simulink model "old_quadSimulinkRetroComp17"  (R2017a)
settings: Solver=FixedStepAuto  StartTime=0.0  StopTime=3  FixedStep=0.005
values from neighbouring files (symbols this model uses):
  d = 2.4*10^-3    (= 0.0024)    [ScrValBackup.m]    (also in corke_plot.m = quad.d)
  dx0 = 0    [ScrValBackup.m]
  dy0 = 0    [ScrValBackup.m]
  dz0 = 0    [ScrValBackup.m]
  g = 9.81    [ScrValBackup.m]
  kr = 0.1    [ScrValBackup.m]
  l = 0.255    [ScrValBackup.m]
  m = 0.5    [ScrValBackup.m]
  p0 = 0    [ScrValBackup.m]
  phi0 = 0    [ScrValBackup.m]
  psi0 = 0.1    [ScrValBackup.m]
  q0 = 0    [ScrValBackup.m]
  r0 = 0.1177    [ScrValBackup.m]
  theta0 = 0    [ScrValBackup.m]
  x0 = 1    [ScrValBackup.m]    (also in corke_dynamics.m = init; corke_plot.m = [])
  x_coeff = A^-1*x_constr    [ScrValBackup.m]
  y0 = 1    [ScrValBackup.m]
  y_coeff = A^-1*y_constr    [ScrValBackup.m]
  z0 = 1    [ScrValBackup.m]
  z_coeff = A^-1*z_constr    [ScrValBackup.m]
undefined symbols (not defined in the file or in its folder): clientID
libraries: aerolibutil x1
settings Model: Creator=gianl  LastModifiedBy=dinies33
settings SolverCC: ZeroCrossAlgorithm=Adaptive  AlgebraicLoopSolver=LineSearch
settings DataIOCC: ReturnWorkspaceOutputs=on
settings OptimizationCC: EfficientMapNaN2IntZero=off
settings DebuggingCC: ReadBeforeWriteMsg=DisableAll  WriteAfterWriteMsg=DisableAll  WriteAfterReadMsg=DisableAll  AlgebraicLoopMsg=error  MaxConsecutiveZCsMsg=none  MaskedZcDiagnostic=none  MultiTaskDSMMsg=none
settings HardwareCC: TargetBitPerLong=64  TargetBitPerPointer=64  TargetBitPerSizeT=64  TargetBitPerPtrDiffT=64  TargetLongLongMode=on  TargetIntDivRoundTo=Zero  TargetEndianess=LittleEndian  TargetWordSize=64  TargetHWDeviceType=MATLAB Host  ProdEqTarget=off
settings ModelReferenceCC: UpdateModelReferenceTargets=IfOutOfDate
settings SFSimCC: SFSimEcho=off
settings CodeAppCC: MaxIdLength=128
settings GRTTargetCC: TargetLangStandard=C89/C90 (ANSI)  CombineOutputUpdateFcns=off  GRTInterface=on

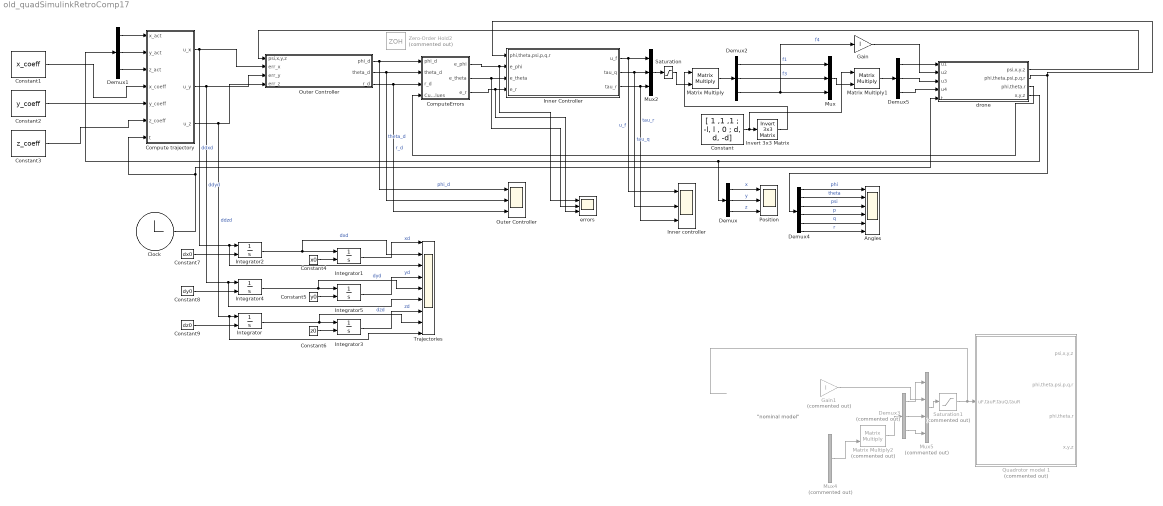
== system old_quadSimulinkRetroComp17 ==
  note: "nominal model"
  Angles : Scope  NumInputPorts=6
  Clock : Clock
  Compute trajectory : MATLAB Function  TreatAsAtomicUnit=on
  "ComputeErrors " : Subsystem
  Constant : Constant  Value=[ 1 ,1 ,1 ; -l, l , 0 ; d, d, -d]
  Constant1 : Constant  Value=x_coeff
  Constant2 : Constant  Value=y_coeff
  Constant3 : Constant  Value=z_coeff
  Constant4 : Constant  Value=x0
  Constant5 : Constant  Value=y0
  Constant6 : Constant  Value=z0
  Constant7 : Constant  Value=dx0
  Constant8 : Constant  Value=dy0
  Constant9 : Constant  Value=dz0
  Demux{,1..2,5} (4 alike) : Demux  Outputs=3
  Demux3 : Demux  Commented=on  Outputs=3
  Demux4 : Demux  Outputs=6
  Gain : Gain  Gain=l
  Gain1 : Gain  Commented=on  Gain=l
  "Inner Controller " : Subsystem
  Inner controller : Scope  NumInputPorts=3
  Integrator{,1..5} (6 alike) : Integrator  InitialConditionSource=external
  Invert 3x3 Matrix : aerolibutil/Invert  3x3 Matrix
  Matrix Multiply : Product  Multiplication=Matrix(*)
  Matrix Multiply1 : Product  Multiplication=Matrix(*)
  Matrix Multiply2 : Product  Commented=on  Multiplication=Matrix(*)
  Mux : Mux  Inputs=3
  Mux2 : Mux  Inputs=3
  Mux4 : Mux  Commented=on  Inputs=3
  Mux5 : Mux  Commented=on
  Outer Controller : Scope  NumInputPorts=3
  "Outer Controller " : Subsystem
  Position : Scope  NumInputPorts=3
  Quadrotor model 1 : Subsystem  Commented=on
  Saturation : Saturate  UpperLimit=40
  Saturation1 : Saturate  Commented=on  UpperLimit=60  LowerLimit=-60
  Trajectories : Scope  NumInputPorts=9
  Zero-Order Hold2 : ZeroOrderHold  Commented=on  SampleTime=0.1
  "drone " : Subsystem
  errors : Scope  NumInputPorts=3
  wires:
  Compute trajectory/3(u_z) -> Trajectories/9, Integrator/1, "Outer Controller "/4(err_z)  "ddzd"
  "drone "/4(x,y,z) -> Demux/1, Demux1/1
  "drone "/1("psi,x,y,z ") -> "Outer Controller "/1(psi,x,y,z)
  "drone "/2("phi,theta,psi,p,q,r ") -> "Inner Controller "/1(phi,theta,psi,p,q,r), Demux4/1
  Compute trajectory/2(u_y) -> Trajectories/6, Integrator4/1, "Outer Controller "/3(err_y)  "ddyd"
  Compute trajectory/1(u_x) -> Trajectories/3, Integrator2/1, "Outer Controller "/2(err_x)  "ddxd"
  "Inner Controller "/1(u_f) -> Inner controller/1, Mux2/1  "u_f"
  "Inner Controller "/3(tau_r) -> Inner controller/3, Mux2/3  "tau_r"
  "Inner Controller "/2(tau_q) -> Inner controller/2, Mux2/2  "tau_q"
  Constant/1 -> Matrix Multiply1/1, Invert 3x3 Matrix/1
  Invert 3x3 Matrix/1 -> Matrix Multiply/1
  Matrix Multiply/1 -> Demux2/1
  "drone "/3("phi,theta,r ") -> "ComputeErrors "/4(Curr_values)
  "ComputeErrors "/1("e_phi ") -> errors/1, "Inner Controller "/2(e_phi)
  Demux2/1 -> Mux/1  "f1"
  Demux2/2 -> Mux/2  "f3"
  Mux2/1 -> Saturation/1
  Demux1/2 -> Compute trajectory/2(y_act)
  Demux1/3 -> Compute trajectory/3(z_act)
  Constant1/1 -> Compute trajectory/4(x_coeff)
  Constant2/1 -> Compute trajectory/5(y_coeff)
  Constant3/1 -> Compute trajectory/6(z_coeff)
  Clock/1 -> "drone "/5(t), Compute trajectory/7(t)
  Demux1/1 -> Compute trajectory/1(x_act)
  "Outer Controller "/1("phi_d ") -> Outer Controller/1, "ComputeErrors "/1(phi_d)  "phi_d"
  Demux3/3 -> Mux5/4
  Mux4/1 -> Matrix Multiply2/2
  ? -> Mux4/2  "f3"
  Mux5/1 -> Saturation1/1
  Demux3/1 -> Mux5/1
  Gain1/1 -> Mux5/2
  ? -> Matrix Multiply2/1
  Saturation1/1 -> Quadrotor model 1/1(uF,tauP,tauQ,tauR)
  Matrix Multiply2/1 -> Demux3/1
  ? -> Gain1/1, Mux4/3  "f4"
  Demux3/2 -> Mux5/3
  ? -> Mux4/1  "f1"
  Integrator2/1 -> Trajectories/2, Integrator1/1  "dxd"
  Integrator1/1 -> Trajectories/1  "xd"
  Integrator/1 -> Trajectories/8, Integrator3/1  "dzd"
  Integrator4/1 -> Trajectories/5, Integrator5/1  "dyd"
  Integrator5/1 -> Trajectories/4  "yd"
  Integrator3/1 -> Trajectories/7  "zd"
  Constant7/1 -> Integrator2/2
  Constant8/1 -> Integrator4/2
  Constant9/1 -> Integrator/2
  Constant5/1 -> Integrator5/2
  Constant4/1 -> Integrator1/2
  Constant6/1 -> Integrator3/2
  "Outer Controller "/2(theta_d) -> Outer Controller/2, "ComputeErrors "/2(theta_d)  "theta_d"
  "Outer Controller "/3(r_d) -> Outer Controller/3, "ComputeErrors "/3(r_d)  "r_d"
  "ComputeErrors "/2(e_theta) -> errors/2, "Inner Controller "/3(e_theta)
  "ComputeErrors "/3(e_r) -> errors/3, "Inner Controller "/4(e_r)
  Demux/2 -> Position/2  "y"
  Demux/1 -> Position/1  "x"
  Demux/3 -> Position/3  "z"
  Demux4/1 -> Angles/1  "phi"
  Demux4/2 -> Angles/2  "theta"
  Demux4/3 -> Angles/3  "psi"
  Demux4/4 -> Angles/4  "p"
  Demux4/5 -> Angles/5  "q"
  Demux4/6 -> Angles/6  "r"
  Saturation/1 -> Matrix Multiply/2
  Demux2/3 -> Gain/1, Mux/3  "f4"
  Mux/1 -> Matrix Multiply1/2
  Demux5/1 -> "drone "/1(u1)
  Demux5/2 -> "drone "/3(u3)
  Demux5/3 -> "drone "/4(u4)
  Matrix Multiply1/1 -> Demux5/1
  Gain/1 -> "drone "/2(u2)

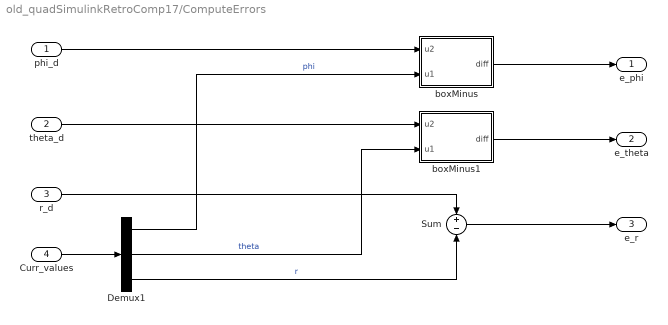
== system old_quadSimulinkRetroComp17/ComputeErrors  ==
  phi_d : Inport
  theta_d : Inport  Port=2
  r_d : Inport  Port=3
  Curr_values : Inport  Port=4
  Demux1 : Demux  Outputs=3
  Sum : Sum  Inputs=+-
  boxMinus : MATLAB Function  TreatAsAtomicUnit=on
  boxMinus1 : MATLAB Function  TreatAsAtomicUnit=on
  "e_phi " : Outport
  e_theta : Outport  Port=2
  e_r : Outport  Port=3
  wires:
  phi_d/1 -> boxMinus/1(u2)
  Demux1/1 -> boxMinus/2(u1)  "phi"
  theta_d/1 -> boxMinus1/1(u2)
  Demux1/2 -> boxMinus1/2(u1)  "theta"
  r_d/1 -> Sum/1
  Demux1/3 -> Sum/2  "r"
  Sum/1 -> e_r/1
  boxMinus1/1(diff) -> e_theta/1
  boxMinus/1(diff) -> "e_phi "/1
  Curr_values/1 -> Demux1/1

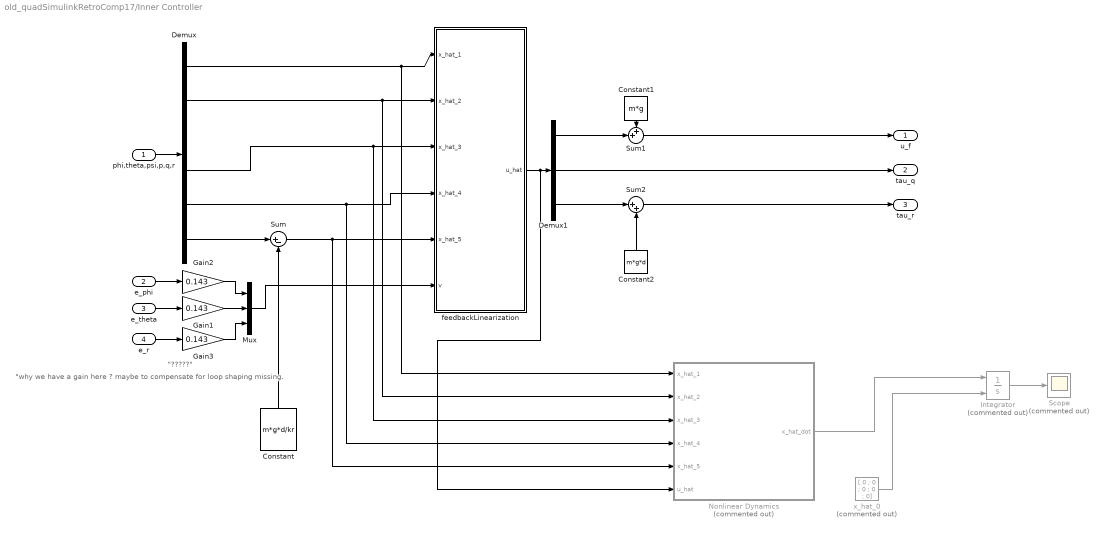
== system old_quadSimulinkRetroComp17/Inner Controller  ==
  note: "why we have a gain here ? maybe to compensate for loop shaping missing.
  note: "?????"
  phi,theta,psi,p,q,r : Inport
  e_phi : Inport  Port=2
  e_theta : Inport  Port=3
  e_r : Inport  Port=4
  Constant : Constant  Value=m*g*d/kr
  Constant1 : Constant  Value=m*g
  Constant2 : Constant  Value=m*g*d
  Demux : Demux  Outputs=6
  Demux1 : Demux  Outputs=3
  Gain1 : Gain  Gain=0.143
  Gain2 : Gain  Gain=0.143
  Gain3 : Gain  Gain=0.143
  Integrator : Integrator  Commented=on  InitialConditionSource=external
  Mux : Mux  Inputs=3
  "Nonlinear Dynamics " : MATLAB Function  Commented=on  TreatAsAtomicUnit=on
  Scope : Scope  Commented=on
  Sum : Sum  Inputs=|+-
  Sum1 : Sum  Inputs=++|
  Sum2 : Sum  Inputs=|++
  feedbackLinearization : MATLAB Function  TreatAsAtomicUnit=on
  x_hat_0 : Constant  Commented=on  Value=[ 0 ; 0 ; 0 ; 0 ; 0]
  u_f : Outport
  tau_q : Outport  Port=2
  tau_r : Outport  Port=3
  wires:
  phi,theta,psi,p,q,r/1 -> Demux/1
  Demux/1 -> feedbackLinearization/1(x_hat_1), "Nonlinear Dynamics "/1(x_hat_1)
  Demux/2 -> feedbackLinearization/2(x_hat_2), "Nonlinear Dynamics "/2(x_hat_2)
  Demux/4 -> "Nonlinear Dynamics "/3(x_hat_3), feedbackLinearization/3(x_hat_3)
  Demux/5 -> feedbackLinearization/4(x_hat_4), "Nonlinear Dynamics "/4(x_hat_4)
  e_phi/1 -> Gain2/1
  "Nonlinear Dynamics "/1(x_hat_dot) -> Integrator/1
  x_hat_0/1 -> Integrator/2
  Demux/6 -> Sum/1
  Constant/1 -> Sum/2
  Sum/1 -> "Nonlinear Dynamics "/5(x_hat_5), feedbackLinearization/5(x_hat_5)
  Demux1/3 -> Sum2/1
  Demux1/1 -> Sum1/2
  Constant1/1 -> Sum1/1
  Sum1/1 -> u_f/1
  Demux1/2 -> tau_q/1
  Constant2/1 -> Sum2/2
  Sum2/1 -> tau_r/1
  feedbackLinearization/1(u_hat) -> "Nonlinear Dynamics "/6(u_hat), Demux1/1
  Integrator/1 -> Scope/1
  e_theta/1 -> Gain1/1
  e_r/1 -> Gain3/1
  Mux/1 -> feedbackLinearization/6(v)
  Gain2/1 -> Mux/1
  Gain1/1 -> Mux/2
  Gain3/1 -> Mux/3

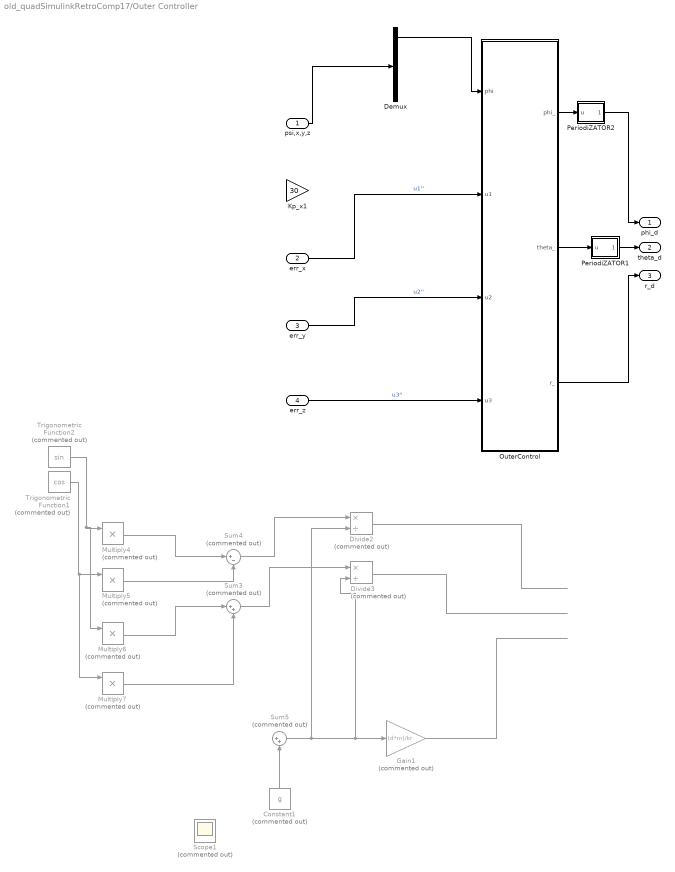
== system old_quadSimulinkRetroComp17/Outer Controller  ==
  psi,x,y,z : Inport  SampleTime=0.1
  err_x : Inport  Port=2
  err_y : Inport  Port=3
  err_z : Inport  Port=4
  Constant1 : Constant  Commented=on  Value=g
  Demux : Demux
  Divide2 : Product  Commented=on  Inputs=*/
  Divide3 : Product  Commented=on  Inputs=*/
  Gain1 : Gain  Commented=on  Gain=(d*m)/kr
  Kp_x1 : Gain  Gain=30
  Multiply{4..7} (4 alike) : Product  Commented=on
  OuterControl : MATLAB Function  TreatAsAtomicUnit=on
  PeriodiZATOR1 : MATLAB Function  TreatAsAtomicUnit=on
  PeriodiZATOR2 : MATLAB Function  TreatAsAtomicUnit=on
  Scope1 : Scope  Commented=on
  Sum3 : Sum  Commented=on  Inputs=|++
  Sum4 : Sum  Commented=on  Inputs=|+-
  Sum5 : Sum  Commented=on  Inputs=|++
  Trigonometric Function1 : Trigonometry  Commented=on  Operator=cos
  Trigonometric Function2 : Trigonometry  Commented=on
  "phi_d " : Outport
  theta_d : Outport  Port=2
  r_d : Outport  Port=3
  wires:
  psi,x,y,z/1 -> Demux/1
  Demux/1 -> OuterControl/1(phi)
  Divide2/1 -> ?
  Divide3/1 -> ?
  Gain1/1 -> ?
  Sum5/1 -> Gain1/1, Divide3/2, Divide2/2
  Constant1/1 -> Sum5/2
  Multiply6/1 -> Sum3/1
  Multiply7/1 -> Sum3/2
  Multiply5/1 -> Sum4/2
  Trigonometric Function1/1 -> Multiply5/1, Multiply7/1
  Trigonometric Function2/1 -> Multiply4/1, Multiply6/1
  Multiply4/1 -> Sum4/1
  ? -> Trigonometric Function2/1
  ? -> Trigonometric Function1/1
  ? -> Scope1/1, Sum5/1  "u3''"
  Sum3/1 -> Divide3/1
  Sum4/1 -> Divide2/1
  ? -> Multiply5/2, Multiply6/2  "u2''"
  ? -> Multiply7/2  "u1''"
  ? -> Multiply4/2  "u1''"
  err_x/1 -> OuterControl/2(u1)  "u1''"
  err_y/1 -> OuterControl/3(u2)  "u2''"
  err_z/1 -> OuterControl/4(u3)  "u3''"
  OuterControl/1(phi_) -> PeriodiZATOR2/1(u)
  OuterControl/2(theta_) -> PeriodiZATOR1/1(u)
  OuterControl/3(r_) -> r_d/1
  PeriodiZATOR2/1(angle) -> "phi_d "/1
  PeriodiZATOR1/1(angle) -> theta_d/1

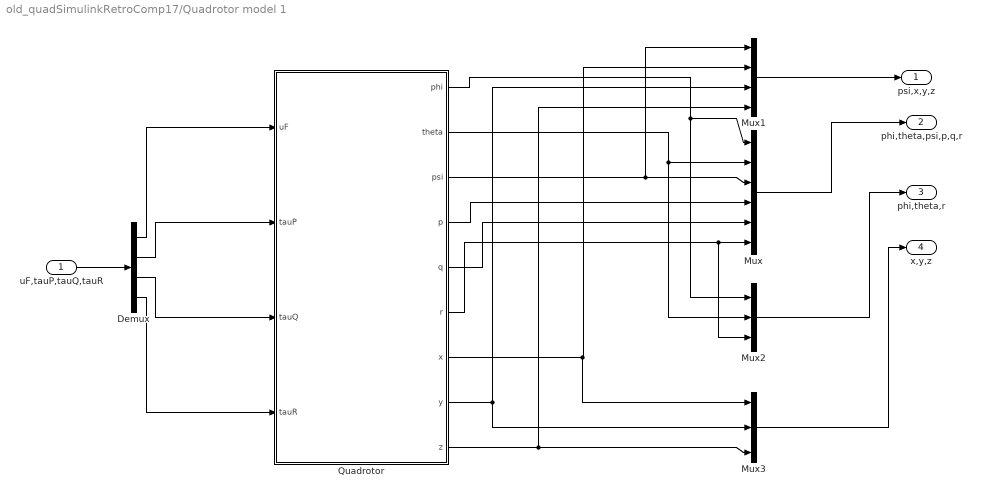
== system old_quadSimulinkRetroComp17/Quadrotor model 1 ==
  uF,tauP,tauQ,tauR : Inport
  Demux : Demux
  Mux : Mux  Inputs=6
  Mux1 : Mux
  Mux2 : Mux  Inputs=3
  Mux3 : Mux  Inputs=3
  "Quadrotor " : Subsystem
  "psi,x,y,z " : Outport
  "phi,theta,psi,p,q,r " : Outport  Port=2
  "phi,theta,r " : Outport  Port=3
  x,y,z : Outport  Port=4
  wires:
  uF,tauP,tauQ,tauR/1 -> Demux/1
  Mux1/1 -> "psi,x,y,z "/1
  Mux/1 -> "phi,theta,psi,p,q,r "/1
  Mux2/1 -> "phi,theta,r "/1
  Mux3/1 -> x,y,z/1
  "Quadrotor "/4(p) -> Mux/4
  "Quadrotor "/5(q) -> Mux/5
  "Quadrotor "/6(r) -> Mux/6, Mux2/3
  "Quadrotor "/7(x) -> Mux3/1, Mux1/2
  "Quadrotor "/8(y) -> Mux1/3, Mux3/2
  "Quadrotor "/9(z) -> Mux1/4, Mux3/3
  Demux/1 -> "Quadrotor "/1(uF)
  Demux/2 -> "Quadrotor "/2(tauP)
  Demux/3 -> "Quadrotor "/3(tauQ)
  Demux/4 -> "Quadrotor "/4(tauR)
  "Quadrotor "/1(phi) -> Mux2/1, Mux/1
  "Quadrotor "/2(theta) -> Mux2/2, Mux/2
  "Quadrotor "/3(psi) -> Mux/3, Mux1/1

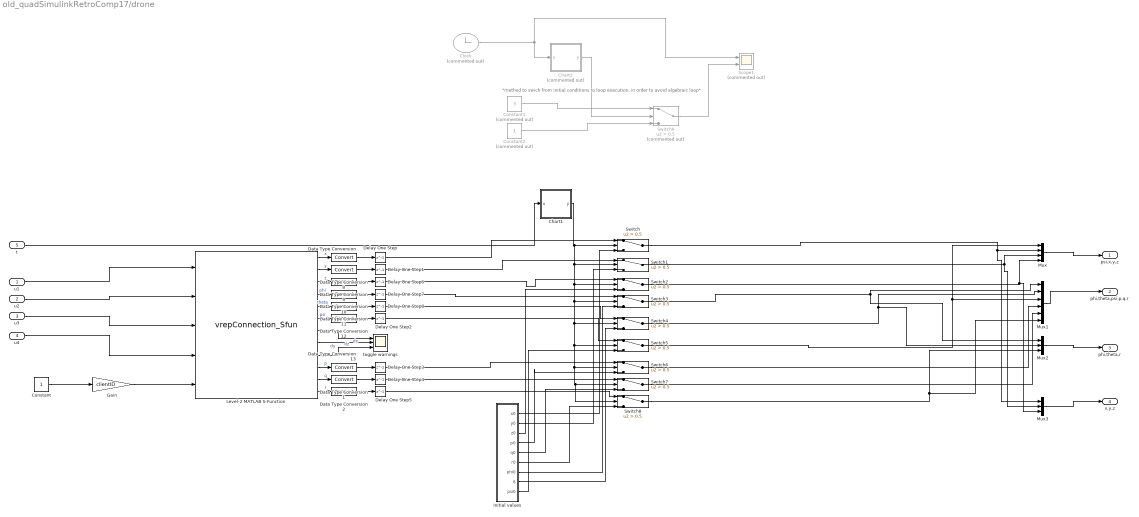
== system old_quadSimulinkRetroComp17/drone  ==
  note: "method to swich from initial conditions to loop execution, in order to avoid algebraic loop"
  u1 : Inport
  u2 : Inport  Port=2
  u3 : Inport  Port=3
  u4 : Inport  Port=4
  t : Inport  Port=5
  Chart1 : Stateflow chart  TreatAsAtomicUnit=on
  Chart2 : Stateflow chart  Commented=on  TreatAsAtomicUnit=on
  Clock : Clock  Commented=on
  Constant : Constant
  Constant1 : Constant  Commented=on  Value=3
  Constant2 : Constant  Commented=on
  Data Type Conversion{,1..2,8..13} (9 alike) : DataTypeConversion
  Delay One Step{,1..8} (9 alike) : Delay  DelayLength=1
  Gain : Gain  Gain=clientID
  "Initial values " : Subsystem
  Level-2 MATLAB S-Function : M-S-Function  FunctionName=vrepConnection_Sfun
  Mux : Mux
  Mux1 : Mux  Inputs=6
  Mux2 : Mux  Inputs=3
  Mux3 : Mux  Inputs=3
  Scope1 : Scope  Commented=on  NumInputPorts=2
  Switch{,1..8} (9 alike) : Switch  Criteria=u2 > Threshold  Threshold=0.5
  Switch9 : Switch  Commented=on  Criteria=u2 > Threshold  Threshold=0.5
  toggle warnings : Scope  NumInputPorts=3
  "psi,x,y,z " : Outport
  "phi,theta,psi,p,q,r " : Outport  Port=2
  "phi,theta,r " : Outport  Port=3
  x,y,z : Outport  Port=4
  wires:
  u1/1 -> Level-2 MATLAB S-Function/1
  u2/1 -> Level-2 MATLAB S-Function/2
  u3/1 -> Level-2 MATLAB S-Function/3
  u4/1 -> Level-2 MATLAB S-Function/4
  Constant/1 -> Gain/1
  Gain/1 -> Level-2 MATLAB S-Function/5
  Level-2 MATLAB S-Function/6 -> Data Type Conversion12/1  "psi"
  Level-2 MATLAB S-Function/5 -> Data Type Conversion11/1  "theta"
  Level-2 MATLAB S-Function/4 -> Data Type Conversion10/1  "phi"
  Level-2 MATLAB S-Function/3 -> Data Type Conversion9/1  "z"
  Level-2 MATLAB S-Function/2 -> Data Type Conversion8/1  "y"
  Level-2 MATLAB S-Function/1 -> Data Type Conversion/1  "x"
  Level-2 MATLAB S-Function/12 -> Data Type Conversion2/1  "r"
  Level-2 MATLAB S-Function/11 -> Data Type Conversion1/1  "q"
  Level-2 MATLAB S-Function/10 -> Data Type Conversion13/1  "p"
  Mux3/1 -> x,y,z/1
  Mux2/1 -> "phi,theta,r "/1
  Mux/1 -> "psi,x,y,z "/1
  Mux1/1 -> "phi,theta,psi,p,q,r "/1
  Switch/1 -> Mux3/1, Mux/2
  Switch1/1 -> Mux3/2, Mux/3
  Switch2/1 -> Mux/4, Mux3/3
  Switch3/1 -> Mux2/1, Mux1/1
  Switch4/1 -> Mux1/2, Mux2/2
  Switch5/1 -> Mux/1, Mux1/3
  Switch6/1 -> Mux1/4
  Switch7/1 -> Mux1/5
  Switch8/1 -> Mux2/3, Mux1/6
  t/1 -> Chart1/1(u)
  Data Type Conversion/1 -> Delay One Step/1
  "Initial values "/1(x0) -> Switch/3
  Data Type Conversion8/1 -> Delay One Step1/1
  "Initial values "/2(y0) -> Switch1/3
  Data Type Conversion9/1 -> Delay One Step6/1
  "Initial values "/3(z0) -> Switch2/3
  Data Type Conversion10/1 -> Delay One Step7/1
  "Initial values "/7(phi0) -> Switch3/3
  "Initial values "/8(theta0) -> Switch4/3
  Data Type Conversion11/1 -> Delay One Step8/1
  Data Type Conversion12/1 -> Delay One Step2/1
  "Initial values "/9(psi0) -> Switch5/3
  Data Type Conversion13/1 -> Delay One Step3/1
  "Initial values "/4(p0) -> Switch6/3
  Data Type Conversion1/1 -> Delay One Step4/1
  "Initial values "/5(q0) -> Switch7/3
  "Initial values "/6(r0) -> Switch8/3
  Data Type Conversion2/1 -> Delay One Step5/1
  Chart2/1(y) -> Switch9/2
  Clock/1 -> Scope1/1, Chart2/1(u)
  Constant1/1 -> Switch9/1
  Switch9/1 -> Scope1/2
  Constant2/1 -> Switch9/3
  Delay One Step5/1 -> Switch8/1
  Delay One Step4/1 -> Switch7/1
  Delay One Step3/1 -> Switch6/1
  Delay One Step2/1 -> Switch5/1
  Delay One Step1/1 -> Switch1/1
  Delay One Step/1 -> Switch/1
  Delay One Step6/1 -> Switch2/1
  Delay One Step7/1 -> Switch3/1
  Delay One Step8/1 -> Switch4/1
  Chart1/1(y) -> Switch3/2, Switch8/2, Switch7/2, Switch6/2, Switch5/2, Switch4/2, Switch2/2, Switch1/2, Switch/2
  Level-2 MATLAB S-Function/7 -> toggle warnings/1  "dx"
  Level-2 MATLAB S-Function/8 -> toggle warnings/2  "dy"
  Level-2 MATLAB S-Function/9 -> toggle warnings/3  "dz"

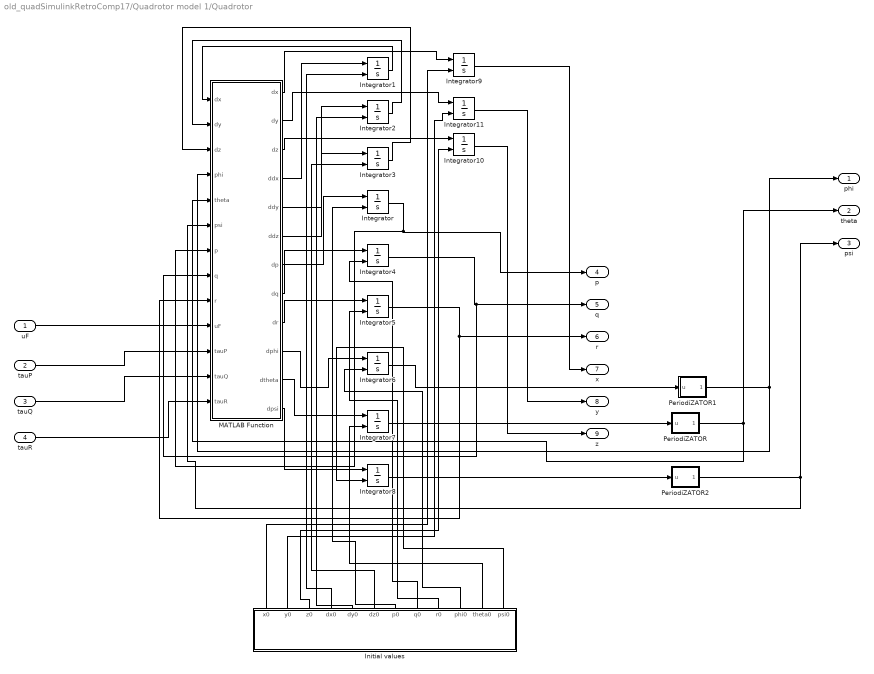
== system old_quadSimulinkRetroComp17/Quadrotor model 1/Quadrotor  ==
  uF : Inport
  tauP : Inport  Port=2
  tauQ : Inport  Port=3
  tauR : Inport  Port=4
  "Initial values " : Subsystem
  Integrator{,1..11} (12 alike) : Integrator  InitialConditionSource=external
  MATLAB Function : MATLAB Function  TreatAsAtomicUnit=on
  PeriodiZATOR : MATLAB Function  TreatAsAtomicUnit=on
  PeriodiZATOR1 : MATLAB Function  TreatAsAtomicUnit=on
  PeriodiZATOR2 : MATLAB Function  TreatAsAtomicUnit=on
  phi : Outport
  theta : Outport  Port=2
  psi : Outport  Port=3
  p : Outport  Port=4
  q : Outport  Port=5
  r : Outport  Port=6
  x : Outport  Port=7
  y : Outport  Port=8
  z : Outport  Port=9
  wires:
  uF/1 -> MATLAB Function/10(uF)
  tauP/1 -> MATLAB Function/11(tauP)
  tauQ/1 -> MATLAB Function/12(tauQ)
  tauR/1 -> MATLAB Function/13(tauR)
  MATLAB Function/12(dpsi) -> Integrator8/1
  Integrator8/1 -> PeriodiZATOR2/1(u)
  MATLAB Function/11(dtheta) -> Integrator7/1
  Integrator7/1 -> PeriodiZATOR/1(u)
  MATLAB Function/10(dphi) -> Integrator6/1
  Integrator6/1 -> PeriodiZATOR1/1(u)
  MATLAB Function/9(dr) -> Integrator5/1
  Integrator5/1 -> MATLAB Function/9(r), r/1
  MATLAB Function/8(dq) -> Integrator4/1
  Integrator4/1 -> MATLAB Function/8(q), q/1
  MATLAB Function/7(dp) -> Integrator/1
  Integrator/1 -> MATLAB Function/7(p), p/1
  MATLAB Function/6(ddz) -> Integrator3/1
  MATLAB Function/5(ddy) -> Integrator2/1
  MATLAB Function/4(ddx) -> Integrator1/1
  Integrator3/1 -> MATLAB Function/3("dz ")
  Integrator2/1 -> MATLAB Function/2("dy ")
  Integrator1/1 -> MATLAB Function/1("dx ")
  Integrator9/1 -> x/1
  Integrator11/1 -> y/1
  Integrator10/1 -> z/1
  "Initial values "/1(x0) -> Integrator9/2
  "Initial values "/2(y0) -> Integrator11/2
  "Initial values "/3(z0) -> Integrator10/2
  "Initial values "/4(dx0) -> Integrator1/2
  "Initial values "/5(dy0) -> Integrator2/2
  "Initial values "/6(dz0) -> Integrator3/2
  "Initial values "/7(p0) -> Integrator/2
  "Initial values "/8(q0) -> Integrator4/2
  "Initial values "/9(r0) -> Integrator5/2
  "Initial values "/10(phi0) -> Integrator6/2
  "Initial values "/11(theta0) -> Integrator7/2
  "Initial values "/12(psi0) -> Integrator8/2
  MATLAB Function/1(dx) -> Integrator9/1
  MATLAB Function/2(dy) -> Integrator11/1
  MATLAB Function/3(dz) -> Integrator10/1
  PeriodiZATOR/1(angle) -> theta/1, MATLAB Function/5(theta)
  PeriodiZATOR1/1(angle) -> phi/1, MATLAB Function/4(phi)
  PeriodiZATOR2/1(angle) -> psi/1, MATLAB Function/6(psi)

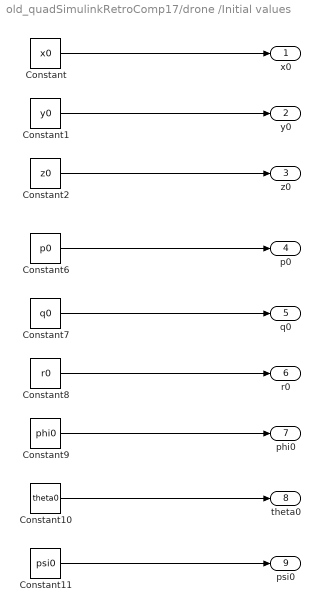
== system old_quadSimulinkRetroComp17/drone /Initial values  ==
  Constant : Constant  Value=x0
  Constant1 : Constant  Value=y0
  Constant10 : Constant  Value=theta0
  Constant11 : Constant  Value=psi0
  Constant2 : Constant  Value=z0
  Constant6 : Constant  Value=p0
  Constant7 : Constant  Value=q0
  Constant8 : Constant  Value=r0
  Constant9 : Constant  Value=phi0
  x0 : Outport
  y0 : Outport  Port=2
  z0 : Outport  Port=3
  p0 : Outport  Port=4
  q0 : Outport  Port=5
  r0 : Outport  Port=6
  phi0 : Outport  Port=7
  theta0 : Outport  Port=8
  psi0 : Outport  Port=9
  wires:
  Constant/1 -> x0/1
  Constant1/1 -> y0/1
  Constant2/1 -> z0/1
  Constant6/1 -> p0/1
  Constant7/1 -> q0/1
  Constant8/1 -> r0/1
  Constant9/1 -> phi0/1
  Constant10/1 -> theta0/1
  Constant11/1 -> psi0/1

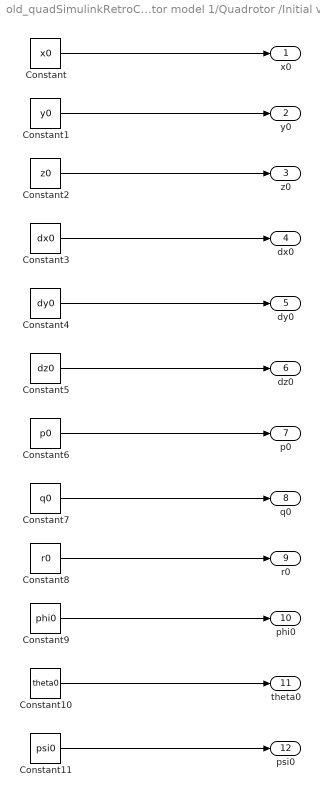
== system old_quadSimulinkRetroComp17/Quadrotor model 1/Quadrotor /Initial values  ==
  Constant : Constant  Value=x0
  Constant1 : Constant  Value=y0
  Constant10 : Constant  Value=theta0
  Constant11 : Constant  Value=psi0
  Constant2 : Constant  Value=z0
  Constant3 : Constant  Value=dx0
  Constant4 : Constant  Value=dy0
  Constant5 : Constant  Value=dz0
  Constant6 : Constant  Value=p0
  Constant7 : Constant  Value=q0
  Constant8 : Constant  Value=r0
  Constant9 : Constant  Value=phi0
  x0 : Outport
  y0 : Outport  Port=2
  z0 : Outport  Port=3
  dx0 : Outport  Port=4
  dy0 : Outport  Port=5
  dz0 : Outport  Port=6
  p0 : Outport  Port=7
  q0 : Outport  Port=8
  r0 : Outport  Port=9
  phi0 : Outport  Port=10
  theta0 : Outport  Port=11
  psi0 : Outport  Port=12
  wires:
  Constant/1 -> x0/1
  Constant1/1 -> y0/1
  Constant2/1 -> z0/1
  Constant3/1 -> dx0/1
  Constant4/1 -> dy0/1
  Constant5/1 -> dz0/1
  Constant6/1 -> p0/1
  Constant7/1 -> q0/1
  Constant8/1 -> r0/1
  Constant9/1 -> phi0/1
  Constant10/1 -> theta0/1
  Constant11/1 -> psi0/1

== matlab function old_quadSimulinkRetroComp17/Inner Controller /feedbackLinearization ==
  data: x_hat_1 input; x_hat_2 input; x_hat_3 input; x_hat_4 input; x_hat_5 input; u_hat output; v input
function u_hat= fcn(x_hat_1,x_hat_2,x_hat_3,x_hat_4,x_hat_5, v)
m= 0.5;
g= 9.81;
d= 1/2; %2.4*10^-3;
kr = 2*10^-3; %extimate for r = 6 (1 rounds /second) 
Ixx= 5.9*10-3;
Iyy= 5.9*10-3;
Izz= 1.16*10-3;
l= 0.255;

x1 = x_hat_1;
x2 = x_hat_2;
x3 = x_hat_3;
x4 = x_hat_4;
x5 = x_hat_5;

alfa = zeros(3,1);

alfa(1,1) = -2*l*Izz*kr^2*(Ixx*(-1/4*cos(x2)^-2*Izz*(2*d^2*g^2*m^2*...
    (sin(2*x1) + x1 + cos(2*x2)*(-4*sin(x1) +x1 ) -sin(2*x2)*x2*tan(x1))+...
    2*d*g*m*kr*( -3*x4 - 4*cos(2*x2)*sin(x1)*x5+ cos(x1)^-1 *(2*x4- ...
    cos(3*x1)*x4 + 2*cos(2*x1)*cos(2*x2)*x4 + sin(3*x1)*x5)+ ...
    (2*sin(2*x2)*x3+ x5)* tan(x1))+ kr^2*( -6*x4*x5 - cos(x1)^-1 *...
    (2 *sin(2*x2)*x3*x4 + 2*cos(3*x1)*x4*x5 + sin(3*x1)*(x4- x5)*(x4+x5))+...
    (x5^2 - 3*x4^2+2*cos(2*x2)*x4^2)*tan(x1))) - cos(x1)^-1*kr^3*x5*tan(x2))+...
    Izz*( kr^2*( cos(x1)^-1 *kr*x5*tan(x2) - d*g*m*( x2+ cos(x1)^-1 *(-1+...
    sin(x1)*x1)*tan(x2)))+Izz*( -kr^2 *x4*x5+d*g*m*kr*(-x4+cos(x1)*x4-...
    sin(x1)*x5+x3*tan(x1)*tan(x2)+ sin(x1)*( x5+ x4*tan(x1))*tan(x2)^2)+...
    d^2 * g^2 * m^2 * (x1- x2*tan(x1)*tan(x2)+ sin(x1)* (-1+ tan(x2)^2)))));

alfa(2,1) =  Izz*kr^2*(Ixx*(-kr^3* x5*tan(x1)+ Izz*( d^2*g^2*m^2*(cos(x1)^-1* ...
    x2 + (-2+cos(x1)) *tan(x2)) + kr^2*(x3*(2*x5+x4*tan(x1))+ cos(x1)^-1*(sin(x1)*...
    x4+ cos(x1)*x5)^2 * tan(x2)) + 2*d*g*m*kr*( x3 - cos(x1)^-1*x3+ (sin(x1)*x4- ...
    x5 +cos(x1)*x5 - x4*tan(x1))* tan(x2)))) + Izz * ( cos(x1)^-1 * kr^2*...
    (d*g*m*( sin(x1) - x1) + sin(x1)*kr*x5) + Izz *(-kr^2*x3*x5+ d^2*g^2*m^2*...
    (-cos(x1)^-1*x2 + tan(x2))+ d*g*m*kr*((-1+ cos(x1)^-1)*x3+(x5+x4*tan(x1))*...
    tan(x2)))));

alfa(3,1) = 0;

% elem 2,2 is dubious, on the paper is written as SCx1, what is S ?
beta = [
    1 , -2*(tan(x1)*tan(x2))/l , -2*(cos(x1)^-1*Ixx*tan(x2))/(l*Izz) ; 
    0 ,  sin(x1)*cos(x1) , Ixx*tan(x1)/Izz ;
    0 ,  0  ,   1;
    ];


u_hat = alfa + beta* v;

== stateflow chart old_quadSimulinkRetroComp17/drone /Chart2 ==
  state ciao
    en, du: y=0;
  state fica
    en, du: y=1;
  ciao -> fica : [u > 0]
  (default) -> ciao
  data: y output; u input

== matlab function old_quadSimulinkRetroComp17/Inner Controller /Nonlinear Dynamics  ==
  data: x_hat_1 input; x_hat_2 input; x_hat_3 input; x_hat_4 input; x_hat_5 input; x_hat_dot output; u_hat input
function x_hat_dot = fcn(x_hat_1,x_hat_2,x_hat_3,x_hat_4,x_hat_5,u_hat)

m= 0.5;
g= 9.81;
d= 2.4*10^-3;
kr = 2*10^-3; %extimate for r = 6 (1 rounds /second) 
Ixx= 5.9*10-3;
Iyy= 5.9*10-3;
Izz= 1.16*10-3;
l= 0.255;
x_hat = [x_hat_1;
        x_hat_2;
        x_hat_3;
        x_hat_4;
        x_hat_5];

f = [
    x_hat(3,1)+x_hat(4,1)*sin(x_hat(1,1))*tan(x_hat(2,1)) + ( x_hat(5,1)+ m*g*d/kr)*cos(x_hat(1,1))*tan(x_hat(2,1));
    x_hat(4,1)*cos(x_hat(1,1))- (x_hat(5,1)+ m*g*d/kr)*sin(x_hat(1,1)) ;
    1/Ixx*( -kr*x_hat(3,1)- x_hat(4,1)*(x_hat(5,1)+ m*g*d/kr)*(Izz - Ixx));
    1/Iyy*( -kr*x_hat(4,1)- x_hat(3,1)*(x_hat(5,1)+ m*g*d/kr)*(Ixx - Izz));
    1/Izz*(-kr* x_hat(5,1));    
    ];
G = [
    0 , 0 , 0;
    0,  0 , 0;
    l/(2*Ixx), 0 , -l/(2*d*Ixx)
    0,  1/Iyy  , 0 ;
    0 ,  0   ,  1/Izz;
    ];

    
x_hat_dot = f + G*u_hat;

== stateflow chart old_quadSimulinkRetroComp17/drone /Chart1 ==
  state ciao
    en, du: y=0;
  state fica
    en, du: y=1;
  ciao -> fica : [u > 0]
  (default) -> ciao
  data: y output; u input

== matlab function old_quadSimulinkRetroComp17/ComputeErrors /boxMinus ==
  data: u2 input; diff output; u1 input
function diff = fcn(u2, u1)

R2 = [cos(u2) -sin(u2);
      sin(u2) cos(u2)];

R1 = [cos(-u1) -sin(-u1);
      sin(-u1) cos(-u1)];

R = R2*R1;

diff = atan2(R(2,1), R(1,1));

== matlab function old_quadSimulinkRetroComp17/ComputeErrors /boxMinus1 ==
  data: u2 input; diff output; u1 input
function diff = fcn(u2, u1)

R2 = [cos(u2) -sin(u2);
      sin(u2) cos(u2)];

R1 = [cos(-u1) -sin(-u1);
      sin(-u1) cos(-u1)];

R = R2*R1;

diff = atan2(R(2,1), R(1,1));

== matlab function old_quadSimulinkRetroComp17/Outer Controller /PeriodiZATOR1 ==
  data: u input; angle output
function angle = fcn(u)

y = sin(u);
x = cos(u);

angle = atan2(y,x);

== matlab function old_quadSimulinkRetroComp17/Outer Controller /PeriodiZATOR2 ==
  data: u input; angle output
function angle = fcn(u)

y = sin(u);
x = cos(u);

angle = atan2(y,x);

== matlab function old_quadSimulinkRetroComp17/Compute trajectory ==
  data: x_act input; y_act input; z_act input; x_coeff input; u_x output; y_coeff input; z_coeff input; u_y output; u_z output; t input
function [u_x, u_y, u_z]  = fcn(x_act, y_act, z_act, x_coeff, y_coeff, z_coeff, t)

x_ = x_coeff(1)*t^3+x_coeff(2)*t^2+x_coeff(3)*t+x_coeff(4);
y_ = y_coeff(1)*t^3+y_coeff(2)*t^2+y_coeff(3)*t+y_coeff(4);
z_ = z_coeff(1)*t^3+z_coeff(2)*t^2+z_coeff(3)*t+z_coeff(4);

x_ddot = 6*x_coeff(1)*t+2*x_coeff(2);
y_ddot = 6*y_coeff(1)*t+2*y_coeff(2);
z_ddot = 6*z_coeff(1)*t+2*z_coeff(2);

u_x = x_ddot + 1.2*(x_ - x_act);
u_y = y_ddot + 0.9*(y_ - y_act);
u_z = z_ddot + 2.3*(z_ - z_act);

== matlab function old_quadSimulinkRetroComp17/Outer Controller /OuterControl ==
  data: phi input; phi_ output; u1 input; u2 input; u3 input; theta_ output; r_ output
function [phi_, theta_, r_] = fcn(phi, u1, u2, u3)

m= 0.5;
g= 9.81;
d= 1/2; %2.4*10^-3;
kr = 1/2; %2*10^-3; %extimate for r = 6 (1 rounds /second) 
l= 0.255;

R = [sin(phi), -cos(phi);
    cos(phi), sin(phi)];


u12 = R*[u1;u2];

u3 = u3 + g;

r_ = u3*d*m/kr;
phi_ = u12(1)/u3;
theta_ = u12(2)/u3;

== matlab function old_quadSimulinkRetroComp17/Quadrotor model 1/Quadrotor /MATLAB Function ==
  data: dx output; dy output; dz output; dx input; dy input; dz input; phi input; theta input; psi input; p input; q input; r input; uF input; ddx output; tauP input; tauQ input; tauR input; ddy output; ddz output; dp output; dq output; dr output; dphi output; dtheta output; dpsi output
function [dx,dy,dz,ddx,ddy,ddz,dp,dq,dr,dphi,dtheta,dpsi] = fcn(dx, dy, dz, phi, theta, psi, p, q, r, uF, tauP, tauQ, tauR)
    
    g = 9.81;
    m = 0.5;
    %l = 0.255;
    %d = 2.4*10^(-3);
    
    kt = 1/2; %2*10^-3;
    kr = 1/2; %2*10^-3;

    Ixx = 5.9*10^(-3);
    Iyy = 5.9*10^(-3);
    Izz = 1.16*10^(-3);

    
    ddx = (1/m)*((cos(phi)*cos(psi)*sin(theta) + sin(phi)*sin(psi))*uF - kt*dx);
    
    ddy = (1/m)*((cos(phi)*sin(theta)*sin(psi) - cos(psi)*sin(phi))*uF - kt*dy);
    
    ddz = (1/m)*((cos(theta)*cos(phi))*uF - m*g - kt*dz);
    
    dp = (1/Ixx)*(-kr*p - q*r*(Izz - Iyy) + tauP);
    
    dq = (1/Iyy)*(-kr*q - p*r*(Ixx - Izz) + tauQ);
    
    dr = (1/Izz)*(-kr*r - p*q*(Iyy - Ixx) + tauR);
    
    dphi = p + q*sin(phi)*tan(phi) + r*cos(phi)*tan(theta);
    
    dtheta = q*cos(phi) - r*sin(phi);
    
    dpsi = (1/cos(theta))*(q*sin(phi) + r*cos(phi));

== matlab function old_quadSimulinkRetroComp17/Quadrotor model 1/Quadrotor /PeriodiZATOR ==
  data: u input; angle output
function angle = fcn(u)

y = sin(u);
x = cos(u);

angle = atan2(y,x);

== matlab function old_quadSimulinkRetroComp17/Quadrotor model 1/Quadrotor /PeriodiZATOR1 ==
  data: u input; angle output
function angle = fcn(u)

y = sin(u);
x = cos(u);

angle = atan2(y,x);

== matlab function old_quadSimulinkRetroComp17/Quadrotor model 1/Quadrotor /PeriodiZATOR2 ==
  data: u input; angle output
function angle = fcn(u)

y = sin(u);
x = cos(u);

angle = atan2(y,x);
